simulink model "s4_3"  (R2018a)
settings: Solver=ode4  StartTime=0.0  StopTime=10.0  FixedStep=0.01  RelTol=1e-3
settings Model: Creator=Filip  LastModifiedBy=Igor
settings DebuggingCC: LibraryContextMissingDiagnostic=warning
settings SFSimCC: SimUseLocalCustomCode=on
settings RTWCC: RTWUseLocalCustomCode=on

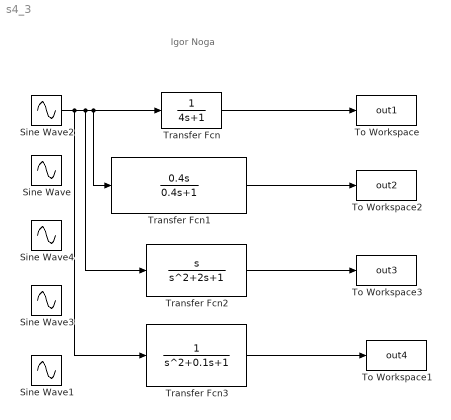
== system s4_3 ==
  note: Igor Noga
  Sine Wave : Sin  Amplitude=3  Phase=5  SampleTime=0
  Sine Wave1 : Sin  Amplitude=4  Frequency=5  SampleTime=0
  Sine Wave2 : Sin  Frequency=0.001  Phase=1  SampleTime=0
  Sine Wave3 : Sin  Amplitude=2  Frequency=0.01  Phase=1  SampleTime=0
  Sine Wave4 : Sin  Frequency=30  Phase=2  SampleTime=0
  To Workspace : ToWorkspace  VariableName=out1  SampleTime=-1
  To Workspace1 : ToWorkspace  VariableName=out4  SampleTime=-1
  To Workspace2 : ToWorkspace  VariableName=out2  SampleTime=-1
  To Workspace3 : ToWorkspace  VariableName=out3  SampleTime=-1
  Transfer Fcn : TransferFcn  Denominator=[4 1]
  Transfer Fcn1 : TransferFcn  Numerator=[0.4 0]  Denominator=[0.4 1]
  Transfer Fcn2 : TransferFcn  Numerator=[1 0]
  Transfer Fcn3 : TransferFcn  Denominator=[1 0.1 1]
  wires:
  Sine Wave2/1 -> Transfer Fcn3/1, Transfer Fcn2/1, Transfer Fcn1/1, Transfer Fcn/1
  Transfer Fcn/1 -> To Workspace/1
  Transfer Fcn1/1 -> To Workspace2/1
  Transfer Fcn2/1 -> To Workspace3/1
  Transfer Fcn3/1 -> To Workspace1/1
